simulink model "double_pendulum_exp"  (R2022a)
settings: Solver=FixedStepAuto  StartTime=0.0  StopTime=10  FixedStep=0.001  RelTol=1e-3  AbsTol=1e-3  EnableMultiTasking=on
libraries: fl_lib x8, nesl_utility x8, sm_lib x7
settings Model: Creator=keonyoung  LastModifiedBy=keonyoung
settings SolverCC: AutoScaleAbsTol=off  AlgebraicLoopSolver=TrustRegion  MaxZcPerStep=1
settings DataIOCC: LimitDataPoints=on  MaxDataPoints=10000
settings OptimizationCC: LifeSpan=inf
settings DebuggingCC: UnconnectedInputMsg=warning  UnconnectedOutputMsg=warning  UnconnectedLineMsg=warning  AllowSymbolicDim=off  SFUnexpectedBacktrackingDiag=warning  SFNoUnconditionalDefaultTransitionDiag=warning  SFExecutionAtInitializationDiag=none  SFMachineParentedDataDiag=warning  ArithmeticOperatorsInVariantConditions=warning
settings SFSimCC: SimUseLocalCustomCode=off  CustomCodeUndefinedFunction=UseInterfaceOnly
settings RTWCC: RTWUseLocalCustomCode=off  DLArmComputeVersion=19.05
settings CodeAppCC: StateflowObjectComments=on
settings GRTTargetCC: TargetLangStandard=C89/C90 (ANSI)
settings ConfigComp: CovMetricSettings=dw  CovSaveCumulativeToWorkspaceVar=on  CovSaveSingleToWorkspaceVar=on  CovExternalEMLEnable=off  CovSFcnEnable=off
settings SimscapeCC: SimscapeLogType=all  SimscapeLogSimulationStatistics=on  SimscapeLogDataHistory=10000

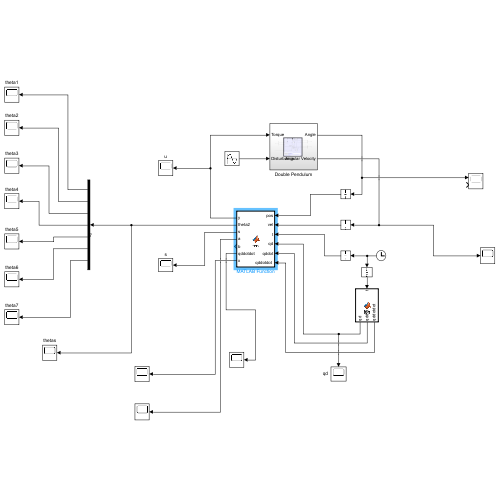
[thumbnail: Simulink's stored preview of the top-level diagram]
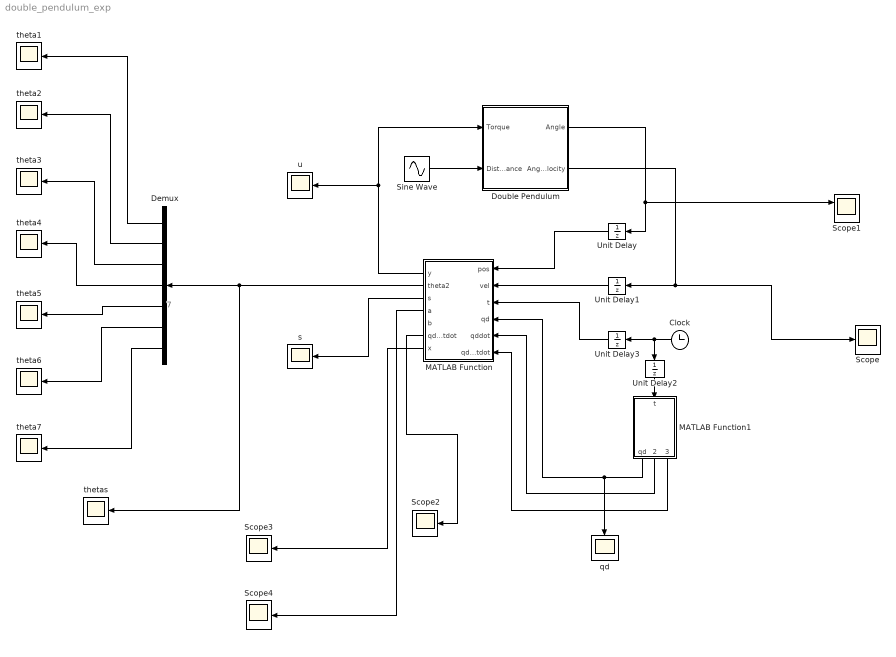
== system double_pendulum_exp ==
  note: 7
  Clock : Clock
  Demux : Demux  Outputs=7
  Double Pendulum : Subsystem
  MATLAB Function : MATLAB Function  TreatAsAtomicUnit=on
  MATLAB Function1 : MATLAB Function  TreatAsAtomicUnit=on
  Scope{,2..4} (4 alike) : Scope
  Scope1 : Scope  NumInputPorts=2
  Sine Wave : Sin  Amplitude=0  Frequency=5  SampleTime=0
  Unit Delay : UnitDelay  SampleTime=-1  HasFrameUpgradeWarning=on
  Unit Delay1 : UnitDelay  InitialCondition=-pi/2  SampleTime=-1  HasFrameUpgradeWarning=on
  Unit Delay2 : UnitDelay  SampleTime=-1  HasFrameUpgradeWarning=on
  Unit Delay3 : UnitDelay  SampleTime=-1  HasFrameUpgradeWarning=on
  qd : Scope
  s : Scope
  theta{1..7} (7 alike) : Scope
  thetas : Scope
  u : Scope
  wires:
  Double Pendulum/1(Angle) -> Unit Delay/1, Scope1/1
  Double Pendulum/2(Angular Velocity) -> Scope/1, Unit Delay1/1
  Unit Delay/1 -> MATLAB Function/1(pos)
  Sine Wave/1 -> Double Pendulum/2(Disturbance)
  Clock/1 -> Unit Delay2/1, Unit Delay3/1
  MATLAB Function/1(y) -> Double Pendulum/1(Torque), u/1
  Unit Delay3/1 -> MATLAB Function/3(t)
  Unit Delay1/1 -> MATLAB Function/2(vel)
  MATLAB Function/3(s) -> s/1
  MATLAB Function1/1(qd) -> qd/1, MATLAB Function/4(qd)
  MATLAB Function1/2(qddot) -> MATLAB Function/5(qddot)
  MATLAB Function1/3(qddotdot) -> MATLAB Function/6("qddotdot ")
  MATLAB Function/2(theta2) -> thetas/1, Demux/1
  Demux/1 -> theta1/1
  Demux/2 -> theta2/1
  Demux/3 -> theta3/1
  Demux/4 -> theta4/1
  Demux/5 -> theta5/1
  Demux/6 -> theta6/1
  Demux/7 -> theta7/1
  MATLAB Function/7(x) -> Scope3/1
  MATLAB Function/6(qddotdot) -> Scope2/1
  Unit Delay2/1 -> MATLAB Function1/1(t)
  MATLAB Function/4(a) -> Scope4/1

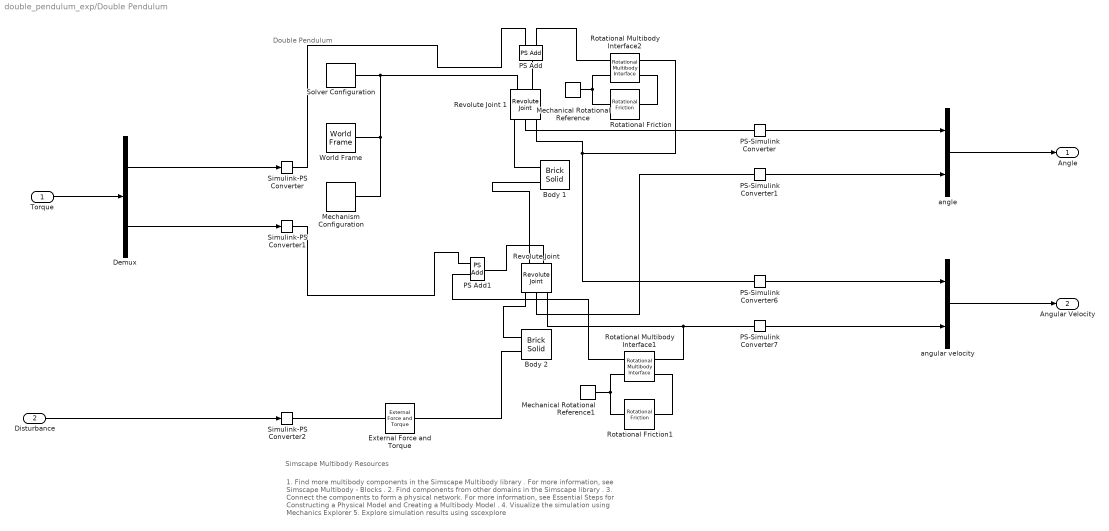
== system double_pendulum_exp/Double Pendulum ==
  note: Double Pendulum
  note: Simscape Multibody Resources
  note: 1. Find more multibody components in the Simscape Multibody library .
      | For more information, see Simscape Multibody - Blocks .
      | 2. Find components from other domains in the Simscape library .
      | 3. Connect the components to form a physical network.
      | For more information, see Essential Steps for Constructing a Physical Model and Creating a Multibody Model .
      | 4. Visualize the simulation using Mechanics Explorer
      | 5. Explore simulation results using sscexplore
  Torque : Inport
  Disturbance : Inport  Port=2
  Body 1 : sm_lib/Body Elements/Brick Solid  GraphicAmbientColor=[0.15 0.15 0.15 1.0]  BasedOnType=Mass  BrickDimensions=[0.269 0.04 0.02]  BrickDimensionUnits=m  CenterOfMass=[0 0 0]  CenterOfMassUnits=m  GraphicDiffuseColor=[0.0 0.4 1.0]  Density=9000  DensityUnits=kg/m^3  DoExposeReferenceFrame=on  GraphicEmissiveColor=[0.0 0.0 0.0 1.0]  ExportEntireGeometry=off  SerializedFrames=<Frames><Frame><Id>Frame1</Id><Value><Name>F1</Name><Origin><Source>GeometricFeature</Source><FeatureName>-x surface</FeatureName></Origin><PrimaryAxis><DefinedDirection>+Z</DefinedDirection><Source>ReferenceFrame</Source><SourceDirection>+Z</SourceDirection><FeatureName></FeatureName></PrimaryAxis><SecondaryAxis><DefinedDirection>+X</DefinedDirection><Source>ReferenceFrame</Source><SourceDirection>+X</SourceDirection><FeatureName></FeatureName></SecondaryAxis></Value></Frame><Frame><Id>Frame2</Id><Value><Name>F2</Name><Origin><Source>GeometricFeature</Source><FeatureName>+x surface</FeatureName></Origin><PrimaryAxis><DefinedDirection>+Z</DefinedDirection><Source>ReferenceFrame</Source><SourceDirection>+Z</SourceDirection><FeatureName></FeatureName></PrimaryAxis><SecondaryAxis><DefinedDirection>+X</DefinedDirection><Source>ReferenceFrame</Source><SourceDirection>+X</SourceDirection><FeatureName></FeatureName></SecondaryAxis></Value></Frame></Frames>  MarkerShape=Sphere  MarkerSize=10  GraphicType=FromGeometry  InertiaType=CalculateFromGeometry  Mass=1.75  MassUnits=kg  MomentsOfInertia=[1 1 1]  MomentsOfInertiaUnits=kg*m^2  GraphicOpacity=1.0  ProductsOfInertia=[0 0 0]  ProductsOfInertiaUnits=kg*m^2  GraphicShininess=75  GraphicSpecularColor=[0.5 0.5 0.5 1.0]  GraphicVisPropType=SimpleVisualProperties
  Body 2 : sm_lib/Body Elements/Brick Solid  GraphicAmbientColor=[0.15 0.15 0.15 1.0]  BasedOnType=Mass  BrickDimensions=[0.343 0.04 0.02]  BrickDimensionUnits=m  CenterOfMass=[0 0 0]  CenterOfMassUnits=m  GraphicDiffuseColor=[1.0 0.2 0.2]  Density=8651  DensityUnits=kg/m^3  DoExposeReferenceFrame=on  GraphicEmissiveColor=[0.0 0.0 0.0 1.0]  ExportEntireGeometry=off  SerializedFrames=<Frames><Frame><Id>Frame1</Id><Value><Name>F1</Name><Origin><Source>GeometricFeature</Source><FeatureName>-x surface</FeatureName></Origin><PrimaryAxis><DefinedDirection>+Z</DefinedDirection><Source>ReferenceFrame</Source><SourceDirection>+Z</SourceDirection><FeatureName></FeatureName></PrimaryAxis><SecondaryAxis><DefinedDirection>+X</DefinedDirection><Source>ReferenceFrame</Source><SourceDirection>+X</SourceDirection><FeatureName></FeatureName></SecondaryAxis></Value></Frame><Frame><Id>Frame2</Id><Value><Name>F2</Name><Origin><Source>GeometricFeature</Source><FeatureName>+x surface</FeatureName></Origin><PrimaryAxis><DefinedDirection>+Z</DefinedDirection><Source>ReferenceFrame</Source><SourceDirection>+Z</SourceDirection><FeatureName></FeatureName></PrimaryAxis><SecondaryAxis><DefinedDirection>+X</DefinedDirection><Source>ReferenceFrame</Source><SourceDirection>+X</SourceDirection><FeatureName></FeatureName></SecondaryAxis></Value></Frame></Frames>  MarkerShape=Sphere  MarkerSize=10  GraphicType=FromGeometry  InertiaType=CalculateFromGeometry  Mass=1.89  MassUnits=kg  MomentsOfInertia=[1 1 1]  MomentsOfInertiaUnits=kg*m^2  GraphicOpacity=1.0  ProductsOfInertia=[0 0 0]  ProductsOfInertiaUnits=kg*m^2  GraphicShininess=75  GraphicSpecularColor=[0.5 0.5 0.5 1.0]  GraphicVisPropType=SimpleVisualProperties
  Demux : Demux  Outputs=2
  External Force and Torque : sm_lib/Forces and Torques/External Force and Torque  ForceResolutionFrame=AttachedFrame  EnableForceX=off  EnableForceY=on  EnableForceZ=off  EnableForce=off  TorqueResolutionFrame=AttachedFrame  EnableTorqueX=off  EnableTorqueY=off  EnableTorqueZ=off  EnableTorque=off
  Mechanical Rotational Reference : fl_lib/Mechanical/Rotational Elements/Mechanical Rotational Reference
      settings: SourceProductBaseCode=PW,SS,VE
  Mechanical Rotational Reference1 : fl_lib/Mechanical/Rotational Elements/Mechanical Rotational Reference
      settings: SourceProductBaseCode=PW,SS,VE
  Mechanism Configuration : sm_lib/Utilities/Mechanism Configuration  UniformGravity=Constant  GravityVector=[0 -9.80665 0]  GravityUnits=m/s^2  LinearizationDelta=0.001  JointModeTransitionNonlinearIterations=2
  PS Add : fl_lib/Physical Signals/Functions/PS Add
      settings: SourceProductBaseCode=PW,SS,VE
  PS Add1 : fl_lib/Physical Signals/Functions/PS Add
      settings: SourceProductBaseCode=PW,SS,VE
  PS-Simulink Converter{,1,6..7} (4 alike) : nesl_utility/PS-Simulink Converter  PhysicalDomain=network_engine_domain  SubClassName=ps_output  LeftPortType=input  RightPortType=output  PseudoPeriodic=off  Frequencies=[]  VectorFormat=inherit  Unit=inherit  AffineConversion=off
      settings: SourceProductBaseCode=SS,PW,VE
  Revolute Joint : sm_lib/Joints/Revolute Joint  JointMode=Normal  SenseConstraintForce=off  SenseConstraintForceX=off  SenseConstraintForceY=off  SenseConstraintForceZ=off  SenseConstraintTorque=off  SenseConstraintTorqueX=off  SenseConstraintTorqueY=off  SenseConstraintTorqueZ=off  SenseTotalForce=off  SenseTotalForceX=off  SenseTotalForceY=off  SenseTotalForceZ=off  SenseTotalTorque=off  SenseTotalTorqueX=off  SenseTotalTorqueY=off  SenseTotalTorqueZ=off  CompositeWrenchDir=FollowerOnBase  CompositeWrenchFrame=BaseFrame  EquilibriumPosition=0  EquilibriumPositionUnits=deg  SpringStiffness=0  SpringStiffnessUnits=N*m/deg  DampingCoefficient=0  DampingCoefficientUnits=N*m/(deg/s)  TorqueActuationMode=InputTorque  MotionActuationMode=ComputedMotion  SensePosition=on  SenseVelocity=on  SenseAcceleration=off  SenseTorqueForce=off  SenseLowerLimitTorqueForce=off  SenseUpperLimitTorqueForce=off  LowerLimitSpecify=off  LowerLimitBound=-90  LowerLimitBoundUnits=deg  LowerLimitStiffness=1e4  LowerLimitStiffnessUnits=N*m/deg  LowerLimitDamping=10  LowerLimitDampingUnits=N*m/(deg/s)  LowerLimitTransitionRegionWidth=0.1  LowerLimitTransitionRegionWidthUnits=deg  UpperLimitSpecify=off  UpperLimitBound=90  UpperLimitBoundUnits=deg  UpperLimitStiffness=1e4  UpperLimitStiffnessUnits=N*m/deg  UpperLimitDamping=10  UpperLimitDampingUnits=N*m/(deg/s)  UpperLimitTransitionRegionWidth=0.1  UpperLimitTransitionRegionWidthUnits=deg  PositionTargetSpecify=on  PositionTargetPriority=High  PositionTargetValue=45  PositionTargetValueUnits=deg  VelocityTargetSpecify=off  VelocityTargetPriority=High  VelocityTargetValue=0  VelocityTargetValueUnits=deg/s
  Revolute Joint 1 : sm_lib/Joints/Revolute Joint  JointMode=Normal  SenseConstraintForce=off  SenseConstraintForceX=off  SenseConstraintForceY=off  SenseConstraintForceZ=off  SenseConstraintTorque=off  SenseConstraintTorqueX=off  SenseConstraintTorqueY=off  SenseConstraintTorqueZ=off  SenseTotalForce=off  SenseTotalForceX=off  SenseTotalForceY=off  SenseTotalForceZ=off  SenseTotalTorque=off  SenseTotalTorqueX=off  SenseTotalTorqueY=off  SenseTotalTorqueZ=off  CompositeWrenchDir=FollowerOnBase  CompositeWrenchFrame=BaseFrame  EquilibriumPosition=0  EquilibriumPositionUnits=deg  SpringStiffness=0  SpringStiffnessUnits=N*m/deg  DampingCoefficient=0  DampingCoefficientUnits=N*m/(deg/s)  TorqueActuationMode=InputTorque  MotionActuationMode=ComputedMotion  SensePosition=on  SenseVelocity=on  SenseAcceleration=off  SenseTorqueForce=off  SenseLowerLimitTorqueForce=off  SenseUpperLimitTorqueForce=off  LowerLimitSpecify=off  LowerLimitBound=-90  LowerLimitBoundUnits=deg  LowerLimitStiffness=1e4  LowerLimitStiffnessUnits=N*m/deg  LowerLimitDamping=10  LowerLimitDampingUnits=N*m/(deg/s)  LowerLimitTransitionRegionWidth=0.1  LowerLimitTransitionRegionWidthUnits=deg  UpperLimitSpecify=off  UpperLimitBound=90  UpperLimitBoundUnits=deg  UpperLimitStiffness=1e4  UpperLimitStiffnessUnits=N*m/deg  UpperLimitDamping=10  UpperLimitDampingUnits=N*m/(deg/s)  UpperLimitTransitionRegionWidth=0.1  UpperLimitTransitionRegionWidthUnits=deg  PositionTargetSpecify=on  PositionTargetPriority=High  PositionTargetValue=-90  PositionTargetValueUnits=deg  VelocityTargetSpecify=off  VelocityTargetPriority=High  VelocityTargetValue=0  VelocityTargetValueUnits=deg/s
  Rotational Friction : fl_lib/Mechanical/Rotational Elements/Rotational Friction  brkwy_trq=1 N*m  brkwy_vel=0.001 rad/s  Col_trq=1 N*m  visc_coef=1 N*m*s/rad  w_specify=off  w_priority=None  w=0 rad/s  w_nominal_specify=off  w_nominal_unit=rad/s  w_nominal_value=1  t_specify=off  t_priority=None  t=0 N*m  t_nominal_specify=off  t_nominal_unit=N*m  t_nominal_value=1
      settings: SourceProductBaseCode=PW,SS,VE
  Rotational Friction1 : fl_lib/Mechanical/Rotational Elements/Rotational Friction  brkwy_trq=1 N*m  brkwy_vel=0.001 rad/s  Col_trq=1 N*m  visc_coef=1 N*m*s/rad  w_specify=off  w_priority=None  w=0 rad/s  w_nominal_specify=off  w_nominal_unit=rad/s  w_nominal_value=1  t_specify=off  t_priority=None  t=0 N*m  t_nominal_specify=off  t_nominal_unit=N*m  t_nominal_value=1
      settings: SourceProductBaseCode=PW,SS,VE
  Rotational Multibody Interface1 : fl_lib/Mechanical/Multibody Interfaces/Rotational Multibody Interface
      settings: SourceProductBaseCode=PW,SS,VE
  Rotational Multibody Interface2 : fl_lib/Mechanical/Multibody Interfaces/Rotational Multibody Interface
      settings: SourceProductBaseCode=PW,SS,VE
  Simulink-PS Converter : nesl_utility/Simulink-PS Converter  PhysicalDomain=network_engine_domain  SubClassName=ps_input  LeftPortType=input  RightPortType=output  PseudoPeriodic=off  Frequencies=[]  NoiseDistribution=none  NoiseParameters=[]  Unit=N*m  AffineConversion=off  FilteringAndDerivatives=provide  SimscapeFilterOrder=1  InputFilterTimeConstant=0.001  UdotUserProvided=0
      settings: SourceProductBaseCode=SS,PW,VE
  Simulink-PS Converter1 : nesl_utility/Simulink-PS Converter  PhysicalDomain=network_engine_domain  SubClassName=ps_input  LeftPortType=input  RightPortType=output  PseudoPeriodic=off  Frequencies=[]  NoiseDistribution=none  NoiseParameters=[]  Unit=N*m  AffineConversion=off  FilteringAndDerivatives=provide  SimscapeFilterOrder=1  InputFilterTimeConstant=0.001  UdotUserProvided=0
      settings: SourceProductBaseCode=SS,PW,VE
  Simulink-PS Converter2 : nesl_utility/Simulink-PS Converter  PhysicalDomain=network_engine_domain  SubClassName=ps_input  LeftPortType=input  RightPortType=output  PseudoPeriodic=off  Frequencies=[]  NoiseDistribution=none  NoiseParameters=[]  Unit=1  AffineConversion=off  FilteringAndDerivatives=provide  SimscapeFilterOrder=1  InputFilterTimeConstant=0.001  UdotUserProvided=0
      settings: SourceProductBaseCode=SS,PW,VE
  Solver Configuration : nesl_utility/Solver Configuration  PhysicalDomain=network_engine_domain  SubClassName=solver  LeftPortType=input  RightPortType=generic  Tones=[]  Harmonics=[]  SimulateNoise=off  Profile=off  UseLocalSampling=off  EnableSwitchedLinearOptims=on  FrequencyDomain=off  UseCCode=off  RelTol=0.001  AbsTol=1e-06  MinStep=1e-09  ToWorkspace=off  RevertToSquareIcSolve=off  NumHomotopyIterations=100  PhasorMode=off  PhasorModeNumHarmonics=1  IndexReductionMethod=DerivativeReplacement  DoDC=on  ResidualTolerance=1e-09  UseLocalSolver=off  LocalSolverChoice=NE_BACKWARD_EULER_ADVANCER  LocalSolverSampleTime=0.001  DoFixedCost=off  MaxNonlinIter=3  MaxModeIter=2  ComputeImpulses=off  ImpulseIterations=2  LinearAlgebra=Sparse  LinearAlgebraNumThread=0  EquationFormulation=NE_TIME_EF  DelaysMemoryBudget=1024  AutomaticFiltering=on  FilteringTimeConstant=0.001  PartitionStorageMethod=AS_NEEDED  PartitionMemoryBudget=1024  PartitionMethod=FAST
      settings: SourceProductBaseCode=SS,PW,VE
  World Frame : sm_lib/Frames and Transforms/World Frame
  angle : Mux  Inputs=2
  angular velocity : Mux  Inputs=2
  Angle : Outport
  Angular Velocity : Outport  Port=2
  wires:
  PS-Simulink Converter/1 -> angle/1
  PS-Simulink Converter1/1 -> angle/2
  PS-Simulink Converter6/1 -> angular velocity/1
  PS-Simulink Converter7/1 -> angular velocity/2
  Torque/1 -> Demux/1
  angle/1 -> Angle/1
  angular velocity/1 -> Angular Velocity/1
  Disturbance/1 -> Simulink-PS Converter2/1
  Demux/1 -> Simulink-PS Converter/1
  Demux/2 -> Simulink-PS Converter1/1
  connections:
  Mechanism Configuration/RConn1 -- Revolute Joint 1/LConn1 -- Solver Configuration/RConn1 -- World Frame/RConn1
  Body 2/LConn2 -- External Force and Torque/RConn1
  Revolute Joint/LConn1 -- Body 1/LConn2
  Revolute Joint/RConn1 -- Body 2/LConn1
  Revolute Joint/RConn3 -- Rotational Multibody Interface1/RConn1 -- PS-Simulink Converter7/LConn1
  Revolute Joint 1/RConn2 -- PS-Simulink Converter/LConn1
  Revolute Joint/RConn2 -- PS-Simulink Converter1/LConn1
  Simulink-PS Converter2/RConn1 -- External Force and Torque/LConn1
  Revolute Joint 1/RConn3 -- Rotational Multibody Interface2/RConn1 -- PS-Simulink Converter6/LConn1
  Revolute Joint 1/RConn1 -- Body 1/LConn1
  PS Add/LConn2 -- Simulink-PS Converter/RConn1
  Simulink-PS Converter1/RConn1 -- PS Add1/LConn1
  Rotational Friction/LConn1 -- Rotational Multibody Interface2/RConn2
  Rotational Friction/RConn1 -- Rotational Multibody Interface2/LConn2 -- Mechanical Rotational Reference/LConn1
  PS Add/LConn1 -- Rotational Multibody Interface2/LConn1
  Rotational Multibody Interface1/LConn2 -- Mechanical Rotational Reference1/LConn1 -- Rotational Friction1/RConn1
  Rotational Multibody Interface1/RConn2 -- Rotational Friction1/LConn1
  Rotational Multibody Interface1/LConn1 -- PS Add1/LConn2
  PS Add/RConn1 -- Revolute Joint 1/LConn2
  PS Add1/RConn1 -- Revolute Joint/LConn2

== matlab function double_pendulum_exp/MATLAB Function1 ==
  data: t input; qd output; qddot output; qddotdot output
function [qd, qddot, qddotdot]= fcn(t)
persistent count;
persistent period;
if isempty(count)
    count = 0;
    period = 1;
end
if t >= 0
    x = t-count;
%     x
%     qd = [((x-8)^3*(x-2)^3*(x)^3)/93312 - pi/2; 0];
%     qddot = [x^2*(x^2-10*x+16)^2*(3*x^2-20*x+16)/31104; 0];
%     qddotdot= [x*(3*x^6-70*x^5+609*x^4-2450*x^3+4640*x^2-3840*x+1024)/3888; 0];
%     qd = [3*x^4*(x-1)*(x-2)^4-pi/2; 3*x^4*(x-1)*(x-2)^4];
%     qddot = [3*(x-2)^3*x^3*(9*x^2-18*x+8); 3*(x-2)^3*x^3*(9*x^2-18*x+8)];
%     qddotdot = [72*(x-2)^2*x^2*(3*x^3-9*x^2+8*x-2); 72*(x-2)^2*x^2*(3*x^3-9*x^2+8*x-2)];
    if period == 1
        qd = [3*(2*x)^4*(2*x-1)*(2*x-2)^4-pi/2; 3*(2*x)^4*(2*x-1)*(2*x-2)^4+pi/4];
        qddot = [1536*(x-1)^3*x^3*(9*x^2-9*x+2); 1536*(x-1)^3*x^3*(9*x^2-9*x+2)];
        qddotdot = [9216*(x-1)^2*x^2*(12*x^3-18*x^2+8*x-1); 9216*(x-1)^2*x^2*(12*x^3-18*x^2+8*x-1)];
    else
        qd = [3*x^4*(x-1)*(x-2)^4-pi/2; 3*x^4*(x-1)*(x-2)^4+pi/4];
        qddot = [3*(x-2)^3*x^3*(9*x^2-18*x+8); 3*(x-2)^3*x^3*(9*x^2-18*x+8)];
        qddotdot = [72*(x-2)^2*x^2*(3*x^3-9*x^2+8*x-2); 72*(x-2)^2*x^2*(3*x^3-9*x^2+8*x-2)];
    end

    if x >= period
        count = count + period;
        if period == 1
            period = 2;
        else
            period = 1;
        end
%         period
    end
else
    qd = [-pi/2; 0];
    qddot = [0; 0];
    qddotdot = [0; 0];
end


%% single frequency

% persistent count;
% if isempty(count)
%     count = 0;
% end
% if t > 1
%     x = t-1;
%     qd = [x^4*(x-1)*(x-3)*(x-5)*(x-7)*(x-9)^4/1000000-pi/2;0];
%     qddot = [((-9+x)^3*x^3*(-945 + 2190*x-1557*x^2+467*x^3-62*x^4+3*x^5))/250000;0];
%     qddotdot = [((-9 + x)^2 *x^2* (25515 - 84510* x + 85395* x^2 - 37674* x^3 + 8109* x^4 - 836* x^5 + 33* x^6))/250000;0];
% else
%     qd = [-pi/2; 0];
%     qddot = [0; 0];
%     qddotdot = [0; 0];
% end

== matlab function double_pendulum_exp/MATLAB Function ==
  settings: updateMethod=DISCRETE
  data: pos input; vel input; t input; y output size=2; theta2 output; s output; a output; b output; qddotdot output; x output; qd input; qddot input; qddotdot input
function [y, theta2, s, a, b, qddotdot, x]= fcn(pos, vel, t, qd, qddot, qddotdot)

%% PID controller
% persistent e_i;
% if isempty(e_i)
%     e_i = [0, 0];
% end
% 
% % pos, vel
% q1 = pos(1);
% q2 = pos(2);
% w1 = vel(1);
% w2 = vel(2);
% 
% Kp1 = 10;
% Ki1 = 0.1;
% Kd1 = 3;
% 
% Kp2 = 10;
% Ki2 = 0.1;
% Kd2 = 3;
% 
% e_i(1) = e_i(1) + (-pi/2-q1)*0.001;
% e_i(2) = e_i(2) + (0-q2)*0.001;
% y = [Kp1*(-pi/2-q1) + Kd1*(0-w1) + Ki1*e_i(1); Kp2*(0-q2) + Kd2*(0-w2) + Ki2*e_i(2), sin(t)];

%% SMC + adaptive controller

% persistent m1;
% persistent m2;
% persistent l1;
% persistent lc1;
% persistent l2;
% persistent lc2;
% persistent I1;
% persistent I2;
% persistent theta;
% persistent gamma;
% persistent lambda;
% 
% if isempty(m1)
%     m1 = 0.2*0.04*0.02*7800;
%     m2 = 0.2*0.04*0.02*7800;
%     l1 = 0.2;
%     lc1 = 0.1;
%     l2 = 0.2;
%     lc2 = 0.1;
%     I1 = 1/12*(4*0.2*0.2+0.04*0.04)*m1;
%     I2 = 1/12*(4*0.2*0.2+0.04*0.04)*m2;
%     theta = [m1*lc1^2+m2*(l1^2+lc2^2)+I1+I2; m2*lc2^2+I2; m2*l1*lc2; m1*lc1+m2*l1; m2*lc2]
%     gamma = [0.001];
%     lambda = [50, 50; 50, 50];
% end
% 
% g = 9.8065;
% q1 = pos(1);
% q2 = pos(2);
% q1dot = vel(1);
% q2dot = vel(2);
% q1dotdot = acc(1);
% q2dotdot = acc(2);
% 
% s = [q1dot+qddot; q2dot-qddot] + 50*[q1-qd; q2-qd];
% 
% Y = [q1dotdot, q2dotdot, (2*q1dotdot + q2dotdot)*cos(q2) - (2*q1dot*q2dot + q2dot^2)*sin(q2), g*cos(q1), g*cos(q1 + q2);
%         0, q1dotdot + q2dotdot, q1dotdot*cos(q2) + (q1dot^2)*sin(q2), 0, g*cos(q1 + q2)];
% 
% theta = theta - 3*transpose(Y)*s*0.001;
% 
% theta2 = theta
% 
% sat_param1 = 10;
% if abs(s(1)) >= sat_param1
%     sat_result1 = sign(s(1));
% else
%     sat_result1 = sign(s(1))*abs(s(1))/sat_param1;
% end
% 
% if abs(s(2)) >= sat_param1
%     sat_result2 = sign(s(2));
% else
%     sat_result2 = sign(s(2))*abs(s(2))/sat_param1;
% end
% 
% % y = Y*theta - 10*[sign(s(1)); sign(s(2))] - [theta(1) + 2*theta(3)*cos(q2), theta(2) + theta(3)*cos(q2); theta(2) + theta(3)*cos(q2), theta(2)]*([q1dotdot+pi/2*cos(t); q2dotdot] + lambda*[q1dot+pi/2*sin(t); q2dot])
% y = Y*theta - 10*[sat_result1; sat_result2] - [theta(1) + 2*theta(3)*cos(q2), theta(2) + theta(3)*cos(q2); theta(2) + theta(3)*cos(q2), theta(2)]*([q1dotdot+pi/2*cos(t); q2dotdot] + lambda*[q1dot+pi/2*sin(t); q2dot]);
% 
% err = [q1-pi/2*cos(t)+pi/2; q2];

%% SMC advanced

persistent m1;
persistent m2;
persistent true_m1;
persistent true_m2;
persistent l1;
persistent lc1;
persistent l2;
persistent lc2;
persistent I1;
persistent I2;
persistent theta;
persistent gamma;
persistent lambda;
persistent true_theta;
persistent true_I1;
persistent true_I2;
persistent K;
persistent d_bound;
if isempty(m1)
    m1 = 0.269*0.04*0.02*7800;
    true_m1 = 1.75;
    m2 = 0.343*0.04*0.02*7800;
    true_m2 = 1.89;
    l1 = 0.269;
    lc1 = 0.1345;
    l2 = 0.343;
    lc2 = 0.1715;
    I1 = 1/12*(4*l1^2+0.04^2)*m1;
    true_I1 = 1/12*(4*l1^2+0.04^2)*true_m1;
    I2 = 1/12*(4*l2^2+0.04^2)*m2;
    true_I2 = 1/12*(4*l2^2+0.04^2)*true_m2;
    theta = [m1*lc1^2+m2*(l1^2+lc2^2)+I1+I2; m2*lc2^2+I2; m2*l1*lc2; m1*lc1+m2*l1; m2*lc2; 0; 0];
%     theta = [m1*lc1^2+m2*(l1^2+lc2^2)+I1+I2; m2*lc2^2+I2; m2*l1*lc2; m1*lc1+m2*l1; m2*lc2];
%     theta = [0;0;0;0;0;0;0];
    true_theta = [true_m1*lc1^2+true_m2*(l1^2+lc2^2)+true_I1+true_I2; true_m2*lc2^2+true_I2; true_m2*l1*lc2; true_m1*lc1+true_m2*l1; true_m2*lc2; 1; 1]
%     true_theta = [true_m1*lc1^2+true_m2*(l1^2+lc2^2)+true_I1+true_I2; true_m2*lc2^2+true_I2; true_m2*l1*lc2; true_m1*lc1+true_m2*l1; true_m2*lc2]
%     theta = true_theta;


%     gamma = 1;
    gamma = [0.5;0.5;0.5;2;2;4;4];
    lambda = 3;    
    K = 10;
    d_bound = 0.001;



end

w1 = pi/2;
w2 = pi/2;
a1 = pi/2;
a2 = pi/6;

g = 9.8065;

input_delay = 0;
if t >= input_delay
  
    q1 = pos(1);
    q2 = pos(2);
    q1dot = vel(1);
    q2dot = vel(2);
%     qd = [a1*(sin(w1*(t-input_delay)))^3-pi/2; a2*(sin(w2*(t-input_delay)))^3];
%     qddot = [3*a1*w1*(sin(w1*(t-input_delay)))^2*cos(w1*(t-input_delay)); 3*a2*w2*(sin(w2*(t-input_delay)))^2*cos(w2*(t-input_delay))];
%     qddotdot = [6*a1*w1^2*sin(w1*(t-input_delay))*(cos(w1*(t-input_delay)))^2-3*a1*w1^2*(sin(w1*(t-input_delay)))^3; 6*a2*w2^2*sin(w2*(t-input_delay))*(cos(w2*(t-input_delay)))^2-3*a2*w2^2*(sin(w2*(t-input_delay)))^3];

else
    q1 = -pi/2;
    q2 = 0;
    q1dot = 0;
    q2dot = 0;
    vel = [0;0];
    pos = [-pi/2;0];
%     qd = [-pi/2;0];
%     qddot = [0;0];
%     qddotdot = [0;0];
end


% declaring s, z, Y %
s = vel-qddot+lambda*(pos-qd); % maybe just multiply scalar??

a  = vel-qddot;
b = pos-qd;

% if t < 2
%     s = (t-1)^2*s;
% end

z = qddotdot-lambda*(vel-qddot);
% z = qddotdot;

Y = [z(1), z(2), (2*z(1) + z(2))*cos(q2) - (2*q1dot*q2dot + q1dot^2)*sin(q2), g*cos(q1), g*cos(q1 + q2), sign(q1dot), q1dot;
        0, z(1) + z(2), z(1)*cos(q2) + (q1dot^2)*sin(q2), 0, g*cos(q1 + q2), sign(q2dot), q2dot];

% Y = [z(1), z(2), (2*z(1) + z(2))*cos(q2) - (2*q1dot*q2dot + q2dot^2)*sin(q2), g*cos(q1), g*cos(q1 + q2);
%         0, z(1) + z(2), z(1)*cos(q2) + (q1dot^2)*sin(q2), 0, g*cos(q1 + q2)];

% dead-zone %
if abs(s(1)) > d_bound
    if abs(s(2)) > d_bound
        update = transpose(Y)*s;
%         update_bound = 20;
%         for i = 1:7
%             if abs(update(i)) >= update_bound
%                 update(i) = update_bound*sign(update(i));
%             end
%         end
        theta = theta - gamma.*update*0.001;
    end
end

% theta = theta - gamma*transpose(Y)*s*0.001;

sat_param1 = 1;

if abs(s(1)) >= sat_param1
    sat_result1 = sign(s(1));
else
    sat_result1 = s(1)/sat_param1;
end

if abs(s(2)) >= sat_param1
    sat_result2 = sign(s(2));
else
    sat_result2 = s(2)/sat_param1;
end

y = Y*theta - K*[sat_result1; sat_result2];
% y = Y*theta - K*s;
% y = Y*theta - K*[sign(s(1)); sign(s(2))];

% if t < 2
%     y = (t-1)*y;
% end

% y = Y*theta - K*s;
x = transpose(Y)*s;
theta2 = theta; 
err = [q1; q2];
